simulink model "spring_mass_damper"  (R2022a)
settings: Solver=ode45  StartTime=0.0  StopTime=100  RelTol=1e-3
settings Model: Creator=Kieran  LastModifiedBy=Kieran

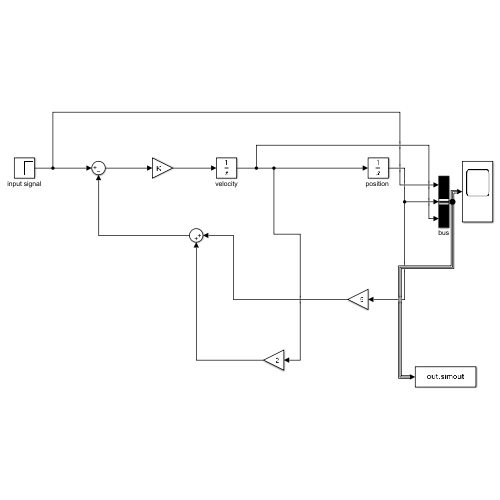
[thumbnail: Simulink's stored preview of the top-level diagram]
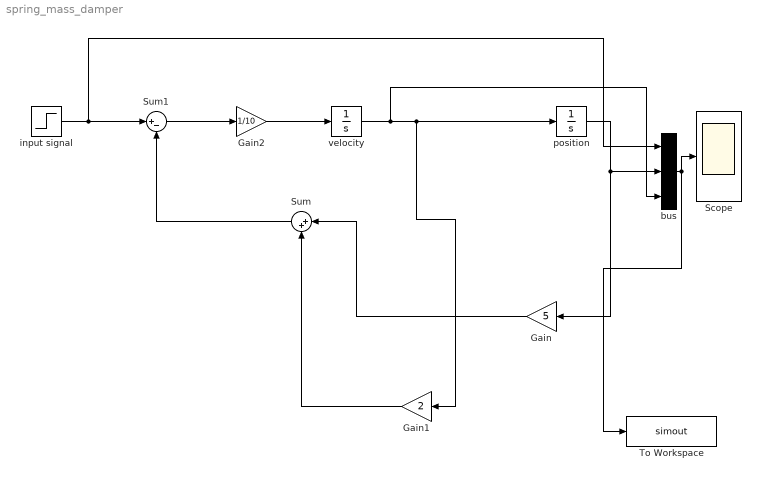
== system spring_mass_damper ==
  Gain : Gain  Gain=5
  Gain1 : Gain  Gain=2
  Gain2 : Gain  Gain=1/10
  Scope : Scope
  Sum : Sum  Inputs=|++
  Sum1 : Sum  Inputs=|+-
  To Workspace : ToWorkspace  VariableName=simout  SaveFormat=Timeseries  SampleTime=-1
  bus : BusCreator  Inputs=3
  input signal : Step  SampleTime=0
  "position " : Integrator
  velocity : Integrator
  wires:
  velocity/1 -> bus/3, Gain1/1, "position "/1
  "position "/1 -> bus/2, Gain/1
  Gain/1 -> Sum/1
  Gain1/1 -> Sum/2
  input signal/1 -> bus/1, Sum1/1
  Sum/1 -> Sum1/2
  Gain2/1 -> velocity/1
  Sum1/1 -> Gain2/1
  bus/1 -> Scope/1, To Workspace/1
